simulink model "Modell"  (R2022b)
settings: Solver=VariableStepAuto  StartTime=0.0  StopTime=1  RelTol=1e-3
values from neighbouring files (symbols this model uses):
  cp = 1.005    [Parameter.m]
  F = 200    [Parameter.m]
  p = 1.225    [Parameter.m]
  T1r = (Td/10)    (= 4.4)    [Parameter.m]
  Taussen = 10    [Parameter.m]
  Th = 0.0014    [Parameter.m]
  Tsoll = 25    [Parameter.m]
  Vh = 5    [Parameter.m]
  Vr = 50    [Parameter.m]
settings Model: Creator=flori  LastModifiedBy=flori

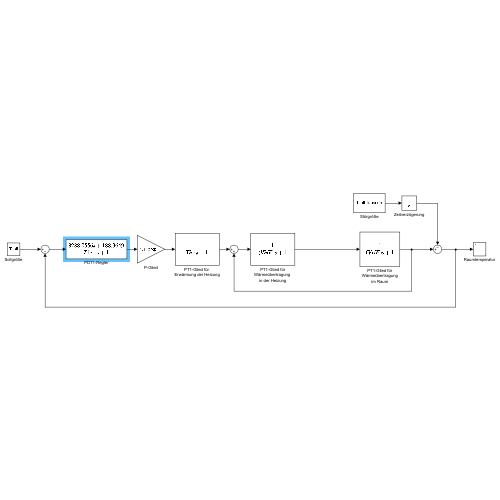
[thumbnail: Simulink's stored preview of the top-level diagram]
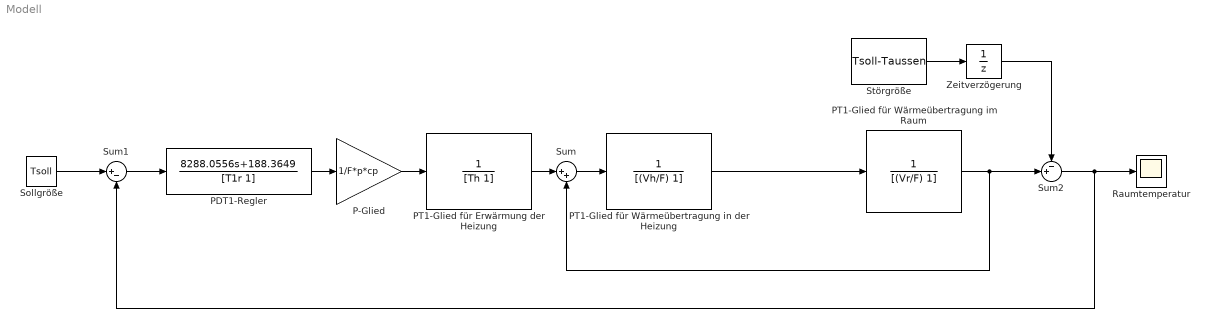
== system Modell ==
  P-Glied : Gain  Gain=1/F*p*cp
  PDT1-Regler : TransferFcn  Numerator=[8288.0556 188.3649]  Denominator=[T1r 1]
  PT1-Glied für Wärmeübertragung im Raum : TransferFcn  Denominator=[(Vr/F) 1]
  PT1-Glied für Wärmeübertragung in der Heizung : TransferFcn  Denominator=[(Vh/F) 1]
  PT1-Glied für Erwärmung der Heizung : TransferFcn  Denominator=[Th 1]
  Raumtemperatur : Scope
  Sollgröße : Constant  Value=Tsoll
  Störgröße : Constant  Value=Tsoll-Taussen  SampleTime=0.5
  Sum : Sum  Inputs=|++
  Sum1 : Sum  Inputs=|+-
  Sum2 : Sum  Inputs=-+|
  Zeitverzögerung : UnitDelay  SampleTime=0.5  HasFrameUpgradeWarning=on
  wires:
  P-Glied/1 -> PT1-Glied für Erwärmung der Heizung/1
  Sollgröße/1 -> Sum1/1
  PT1-Glied für Erwärmung der Heizung/1 -> Sum/1
  Sum/1 -> PT1-Glied für Wärmeübertragung in der Heizung/1
  PT1-Glied für Wärmeübertragung in der Heizung/1 -> PT1-Glied für Wärmeübertragung im Raum/1
  Sum1/1 -> PDT1-Regler/1
  PDT1-Regler/1 -> P-Glied/1
  PT1-Glied für Wärmeübertragung im Raum/1 -> Sum2/2, Sum/2
  Sum2/1 -> Sum1/2, Raumtemperatur/1
  Störgröße/1 -> Zeitverzögerung/1
  Zeitverzögerung/1 -> Sum2/1
